simulink model "GHV_open_att_ang_trajectory_design_equation"  (R2023b)
settings: Solver=VariableStepAuto  StartTime=0.0  StopTime=130  FixedStep=0.0000001  MaxStep=0.1  RelTol=1e-3
undefined symbols (not defined in the file or in its folder): GHV_cfg
libraries: simulink_extras x2
settings Model: SimulationMode=accelerator  Creator=Admin  LastModifiedBy=Admin

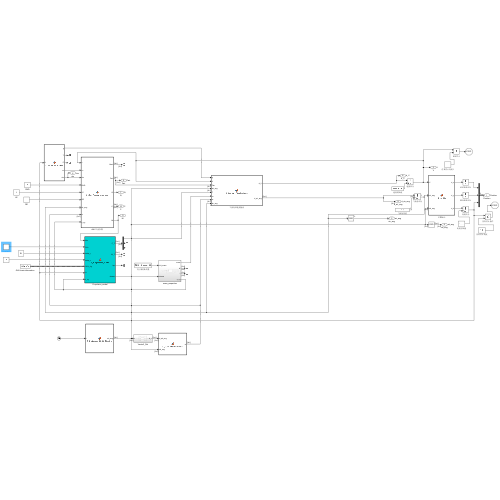
[thumbnail: Simulink's stored preview of the top-level diagram]
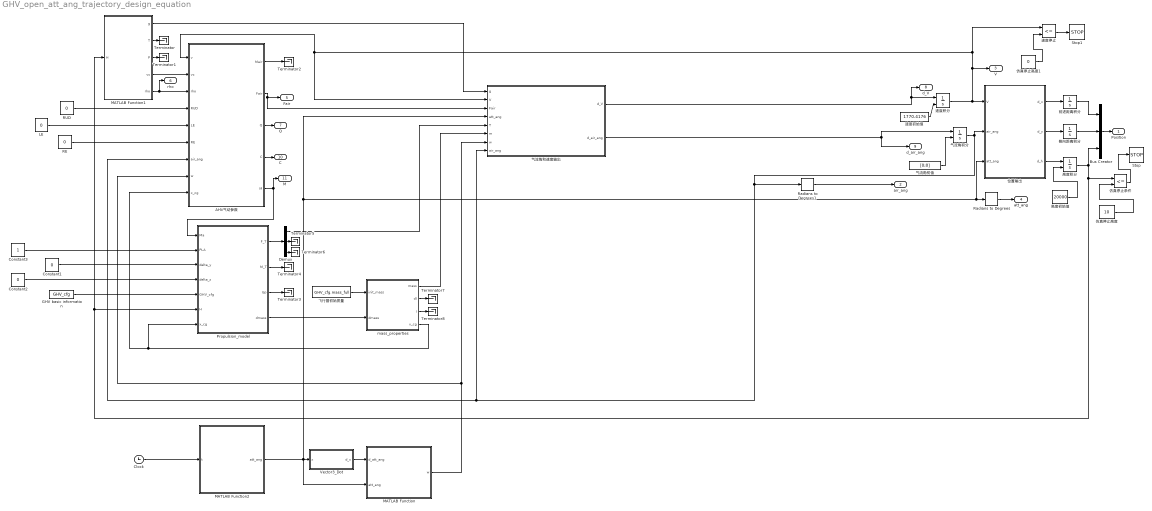
== system GHV_open_att_ang_trajectory_design_equation ==
  AHV气动参数 : MATLAB Function  TreatAsAtomicUnit=on
  Bus Creator : BusCreator  Inputs=3
  Clock : Clock
  Constant1 : Constant  Value=0
  Constant2 : Constant  Value=0
  Constant3 : Constant
  Demux : Demux  Outputs=3
  GHV basic information : Constant  Value=GHV_cfg  VectorParams1D=off  OutDataTypeStr=Bus: slBus1
  LE : Constant  Value=0
  MATLAB Function : MATLAB Function  TreatAsAtomicUnit=on
  MATLAB Function1 : MATLAB Function  TreatAsAtomicUnit=on
  MATLAB Function2 : MATLAB Function  TreatAsAtomicUnit=on
  Propulsion_model : MATLAB Function  TreatAsAtomicUnit=on
  RE : Constant  Value=0
  RUD : Constant  Value=0
  Radians to Degrees : simulink_extras/Transformations/Radians to Degrees
  Radians to Degrees1 : simulink_extras/Transformations/Radians to Degrees
  Stop : Stop
  Stop1 : Stop
  Terminator{,1..8} (9 alike) : Terminator
  Vector3_Dot : Subsystem
  mass_properties : Subsystem
  仿真停止条件 : RelationalOperator  Operator=<=  OutDataTypeStr=boolean  RndMeth=Simplest  InputSameDT=off
  仿真停止高度 : Constant  Value=10
  仿真停止高度1 : Constant  Value=0
  位置输出 : MATLAB Function  TreatAsAtomicUnit=on
  侧向距离积分 : Integrator
  前进距离积分 : Integrator
  气流角初值 : Constant  Value=[0;0]
  气流角和速度输出 : MATLAB Function  TreatAsAtomicUnit=on
  气流角积分 : Integrator  InitialConditionSource=external  InitialCondition=[0;0]
  速度停止 : RelationalOperator  Operator=<=  OutDataTypeStr=boolean  RndMeth=Simplest  InputSameDT=off
  速度初始值 : Constant  Value=1770.4176
  速度积分 : Integrator  InitialConditionSource=external  InitialCondition=2*340
  飞行器初始质量 : Constant  Value=GHV_cfg.mass_full
  高度初始值 : Constant  Value=20000
  高度积分 : Integrator  InitialConditionSource=external  InitialCondition=80000
  Position : Outport  SignalName=Position
  air_ang : Outport  Port=2  SignalName=air_ang
  V : Outport  Port=3  SignalName=V
  att_ang : Outport  Port=4  SignalName=att_ang
  Fair : Outport  Port=5  SignalName=Fair
  rho : Outport  Port=6  SignalName=rho
  Q : Outport  Port=7  SignalName=Q
  d_V : Outport  Port=8  SignalName=d_V
  d_air_ang : Outport  Port=9  SignalName=d_air_ang
  C : Outport  Port=10  SignalName=C
  M : Outport  Port=11
  wires:
  MATLAB Function2/1(att_ang) -> MATLAB Function/2(att_ang), 位置输出/3(att_ang), Radians to Degrees/1, 气流角和速度输出/4(att_ang), Vector3_Dot/1(x)
  气流角积分/1 -> 位置输出/2(air_ang), 气流角和速度输出/8(air_ang), AHV气动参数/7(air_ang), Radians to Degrees1/1
  气流角和速度输出/1(d_V) -> d_V/1, 速度积分/1
  AHV气动参数/2(Fair) -> 气流角和速度输出/3(Fair), Fair/1
  MATLAB Function1/5(rho) -> rho/1, AHV气动参数/3(rho)
  MATLAB Function1/4(vc) -> AHV气动参数/2(vc)
  MATLAB Function1/1(g) -> 气流角和速度输出/1(g)
  位置输出/1(d_x) -> 前进距离积分/1
  位置输出/2(d_y) -> 侧向距离积分/1
  位置输出/3(d_h) -> 高度积分/1
  侧向距离积分/1 -> Bus Creator/2
  前进距离积分/1 -> Bus Creator/1
  Bus Creator/1 -> Position/1
  Radians to Degrees/1 -> att_ang/1
  Radians to Degrees1/1 -> air_ang/1
  RUD/1 -> AHV气动参数/4(RUD)
  仿真停止条件/1 -> Stop/1
  高度积分/1 -> 仿真停止条件/1, Propulsion_model/6(H), MATLAB Function1/1(H), Bus Creator/3
  AHV气动参数/5(M) -> Propulsion_model/1(Ma), M/1
  高度初始值/1 -> 高度积分/2
  速度初始值/1 -> 速度积分/2
  仿真停止高度/1 -> 仿真停止条件/2
  AHV气动参数/3(Q) -> Q/1
  速度积分/1 -> V/1, 速度停止/1, 气流角和速度输出/2(V), AHV气动参数/1(v), 位置输出/1(V)
  仿真停止高度1/1 -> 速度停止/2
  速度停止/1 -> Stop1/1
  气流角和速度输出/2(d_air_ang) -> d_air_ang/1, 气流角积分/1
  AHV气动参数/4(C) -> C/1
  RE/1 -> AHV气动参数/6(RE)
  LE/1 -> AHV气动参数/5(LE)
  气流角初值/1 -> 气流角积分/2
  MATLAB Function/1(w) -> AHV气动参数/8(w), 气流角和速度输出/7(w)
  Clock/1 -> MATLAB Function2/1(t)
  Vector3_Dot/1(d_x) -> MATLAB Function/1(d_att_ang)
  MATLAB Function1/2(T) -> Terminator/1
  MATLAB Function1/3(P) -> Terminator1/1
  飞行器初始质量/1 -> mass_properties/1(init_mass)
  Propulsion_model/4(dmass) -> mass_properties/2(dmass)
  Propulsion_model/3(Isp) -> Terminator3/1
  Propulsion_model/2(M_T) -> Terminator4/1
  mass_properties/1(mass) -> 气流角和速度输出/6(m)
  Propulsion_model/1(F_T) -> Demux/1
  Demux/2 -> Terminator5/1
  Demux/3 -> Terminator6/1
  Demux/1 -> 气流角和速度输出/5(T)
  mass_properties/4(x_cg) -> Propulsion_model/7(x_cg), AHV气动参数/9(x_cg)
  mass_properties/2(dI) -> Terminator7/1
  mass_properties/3(I) -> Terminator8/1
  GHV basic information/1 -> Propulsion_model/5(GHV_cfg)
  Constant2/1 -> Propulsion_model/4(delta_z)
  Constant1/1 -> Propulsion_model/3(delta_y)
  AHV气动参数/1(Mair) -> Terminator2/1
  Constant3/1 -> Propulsion_model/2(PLA)

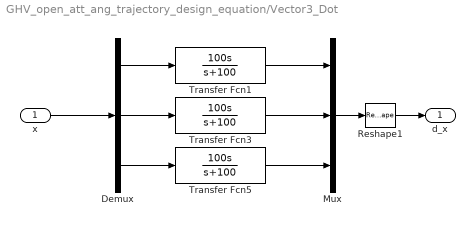
== system GHV_open_att_ang_trajectory_design_equation/Vector3_Dot ==
  x : Inport
  Demux : Demux  Outputs=3
  Mux : Mux  Inputs=3
  Reshape1 : Reshape  OutputDimensionality=Column vector (2-D)
  Transfer Fcn1 : TransferFcn  Numerator=[100 0]  Denominator=[1 100]
  Transfer Fcn3 : TransferFcn  Numerator=[100 0]  Denominator=[1 100]
  Transfer Fcn5 : TransferFcn  Numerator=[100 0]  Denominator=[1 100]
  d_x : Outport
  wires:
  x/1 -> Demux/1
  Demux/2 -> Transfer Fcn3/1
  Demux/1 -> Transfer Fcn1/1
  Demux/3 -> Transfer Fcn5/1
  Mux/1 -> Reshape1/1
  Reshape1/1 -> d_x/1
  Transfer Fcn1/1 -> Mux/1
  Transfer Fcn3/1 -> Mux/2
  Transfer Fcn5/1 -> Mux/3

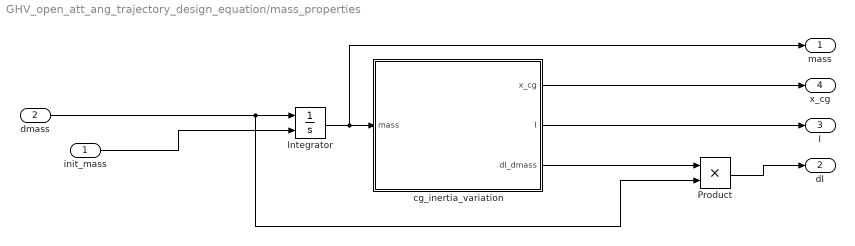
== system GHV_open_att_ang_trajectory_design_equation/mass_properties ==
  init_mass : Inport
  dmass : Inport  Port=2
  Integrator : Integrator  InitialConditionSource=external
  Product : Product
  cg_inertia_variation : MATLAB Function  TreatAsAtomicUnit=on
  mass : Outport
  dI : Outport  Port=2
  I : Outport  Port=3
  x_cg : Outport  Port=4
  wires:
  Integrator/1 -> mass/1, cg_inertia_variation/1(mass)
  init_mass/1 -> Integrator/2
  cg_inertia_variation/3(dI_dmass) -> Product/1
  dmass/1 -> Product/2, Integrator/1
  cg_inertia_variation/2(I) -> I/1
  cg_inertia_variation/1(x_cg) -> x_cg/1
  Product/1 -> dI/1

== matlab function GHV_open_att_ang_trajectory_design_equation/mass_properties/cg_inertia_variation ==
  data: mass input; x_cg output; I output; dI_dmass output
function [x_cg, I, dI_dmass] = S_cg_inertia_variation(mass)

     [x_cg, I, dI_dmass] = cg_inertia_variation(mass);
     
end

== matlab function GHV_open_att_ang_trajectory_design_equation/MATLAB Function2 ==
  data: t input; att_ang output
function att_ang = S_Reference_Flight_Timeline(t)
    att_ang = zeros(3, 1); %#ok<PREALL>
    att_ang = Reference_Flight_Timeline(t);

end

== matlab function GHV_open_att_ang_trajectory_design_equation/MATLAB Function ==
  data: d_att_ang input; w output; att_ang input
function w = S_EulerRate2BodyRate(d_att_ang, att_ang)
    w = zeros(3, 1); %#ok<PREALL>
    w = EulerRate2BodyRate(d_att_ang, att_ang);

end

== matlab function GHV_open_att_ang_trajectory_design_equation/气流角和速度输出 ==
  data: g input; V input; Fair input; att_ang input; T input; m input; w input; air_ang input; d_V output; d_air_ang output
function [d_V, d_air_ang] = S_tra_dyn_VarialbeMass(g, V, Fair, att_ang, T, m, w, air_ang)

     d_V = zeros(1, 1);
     d_air_ang = zeros(2, 1);
    [d_V, d_air_ang] = tra_dyn_VarialbeMass(Fair, T, g, V, air_ang, att_ang, w, m);



end

== matlab function GHV_open_att_ang_trajectory_design_equation/AHV气动参数 ==
  data: Mair output; Fair output; Q output; C output; M output; v input; vc input; rho input; RUD input; LE input; RE input; air_ang input; w input; x_cg input
function [Mair, Fair, Q, C, M] = S_Get_Aerodynamic_xcg(v, vc, rho, RUD, LE, RE, air_ang, w, x_cg)

    Fair = zeros(3, 1);
    Mair = zeros(3, 1);
    C = zeros(6, 1);
    M = zeros(1, 1);
    Q = zeros(1, 1);

[M, Fair, Mair, Q, C] = Get_Aerodynamic_xcg(LE, RE, RUD, air_ang, v, w, vc, rho, x_cg);
   
end

== matlab function GHV_open_att_ang_trajectory_design_equation/MATLAB Function1 ==
  data: g output; H input; T output; P output; vc output; rho output
function [g, T, P, vc, rho] = S_EarthEnvironment(H)

[T, vc, P, rho, g] = EarthEnvironment(H);

end

== matlab function GHV_open_att_ang_trajectory_design_equation/位置输出 ==
  data: V input; d_x output; air_ang input; att_ang input; d_y output; d_h output
function [d_x, d_y, d_h] = S_tra_kin(V, air_ang, att_ang)

   [d_x, d_y, d_h] = tra_kin(V, air_ang, att_ang);

end

== matlab function GHV_open_att_ang_trajectory_design_equation/Propulsion_model ==
  data: Ma input; PLA input; delta_y input; delta_z input; GHV_cfg input; H input; F_T output; M_T output; x_cg input; Isp output; dmass output
function [F_T,M_T, Isp,  dmass] = S_Propulsion_model(Ma, PLA, delta_y, delta_z, GHV_cfg, H, x_cg)
    F_T = zeros(3, 1); %#ok<PREALL>
    M_T = zeros(3, 1); %#ok<PREALL>
   [F_T, M_T, Isp, dmass] = Propulsion_model(PLA, H, Ma, delta_y, delta_z, GHV_cfg, x_cg);

end
